simulink model "Task3_2"  (R2022a)
settings: Solver=FixedStepAuto  StartTime=0.0  StopTime=2  FixedStep=0.00001  RelTol=1e-3
values from neighbouring files (symbols this model uses):
  J_motor = 0.000610871894223    [var_10.mat]
  L_phase = 0.00332259990587    [var_10.mat]
  psi = 0.0961787034043    [var_10.mat]
  R_phase = 0.753894801324    [var_10.mat]
  U_nom = 48    [var_10.mat]
undefined symbols (not defined in the file or in its folder): Ki_i, Kp_i, Kp_W
settings Model: Creator=Family  LastModifiedBy=Family

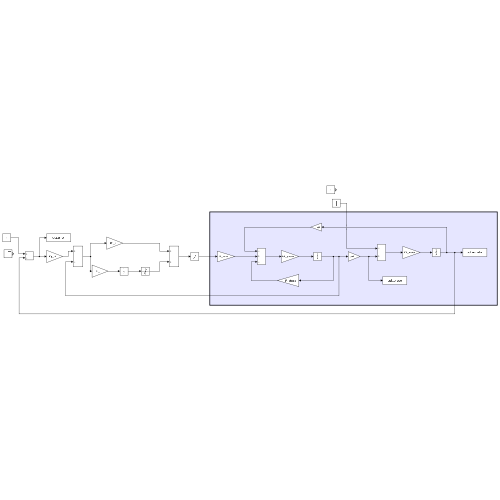
[thumbnail: Simulink's stored preview of the top-level diagram]
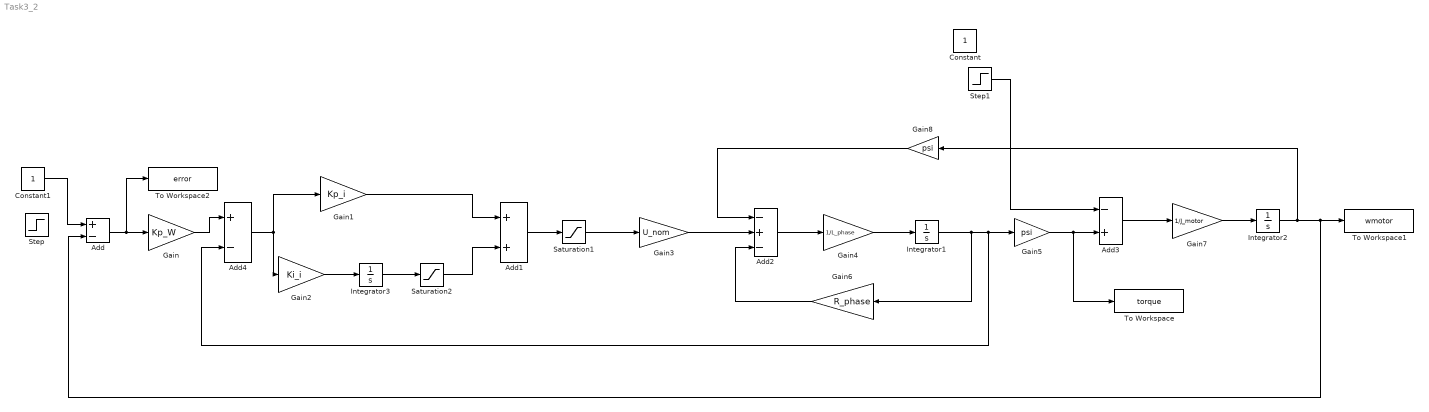
== system Task3_2 ==
  Add : Sum  Inputs=+-
  Add1 : Sum
  Add2 : Sum  Inputs=-+-
  Add3 : Sum  Inputs=-+
  Add4 : Sum  Inputs=+-
  Constant : Constant
  Constant1 : Constant
  Gain : Gain  Gain=Kp_W
  Gain1 : Gain  Gain=Kp_i
  Gain2 : Gain  Gain=Ki_i
  Gain3 : Gain  Gain=U_nom
  Gain4 : Gain  Gain=1/L_phase
  Gain5 : Gain  Gain=psi
  Gain6 : Gain  Gain=R_phase
  Gain7 : Gain  Gain=1/J_motor
  Gain8 : Gain  Gain=psi
  Integrator1 : Integrator
  Integrator2 : Integrator
  Integrator3 : Integrator
  Saturation1 : Saturate  UpperLimit=1  LowerLimit=-1
  Saturation2 : Saturate  UpperLimit=1  LowerLimit=-1
  Step : Step  SampleTime=0
  Step1 : Step  SampleTime=0
  To Workspace : ToWorkspace  VariableName=torque  SaveFormat=Timeseries  SampleTime=0.001
  To Workspace1 : ToWorkspace  VariableName=wmotor  SaveFormat=Timeseries  SampleTime=0.001
  To Workspace2 : ToWorkspace  VariableName=error  SaveFormat=Timeseries  SampleTime=0.001
  wires:
  Gain1/1 -> Add1/1
  Add1/1 -> Saturation1/1
  Gain2/1 -> Integrator3/1
  Add3/1 -> Gain7/1
  Integrator2/1 -> Add/2, To Workspace1/1, Gain8/1
  Gain7/1 -> Integrator2/1
  Step1/1 -> Add3/1
  Gain6/1 -> Add2/3
  Gain5/1 -> To Workspace/1, Add3/2
  Gain4/1 -> Integrator1/1
  Add2/1 -> Gain4/1
  Gain3/1 -> Add2/2
  Integrator1/1 -> Gain6/1, Add4/2, Gain5/1
  Gain8/1 -> Add2/1
  Saturation1/1 -> Gain3/1
  Integrator3/1 -> Saturation2/1
  Saturation2/1 -> Add1/2
  Add4/1 -> Gain2/1, Gain1/1
  Gain/1 -> Add4/1
  Add/1 -> To Workspace2/1, Gain/1
  Constant1/1 -> Add/1
